simulink model "quad_equation_3d_porovnani_modelu_2024a"  (R2024a)
settings: Solver=FixedStepAuto  StartTime=0.0  StopTime=1  FixedStep=0.01  RelTol=1e-3
values from neighbouring files (symbols this model uses):
  b_moment = 0.01    [quad_param_3d.m]
  g = 9.81    [quad_param_3d.m]
  I = [Ixx, 0, 0 ... (first row only)    [quad_param_3d.m]
  Ixx = 1.1    [quad_param_3d.m]
  Iyy = 2.989    [quad_param_3d.m]
  Izz = 3.978    [quad_param_3d.m]
  k = 0.01    [quad_param_3d.m]
  k_thrust = 0.1    [quad_param_3d.m]
  L = 0.086    [quad_param_3d.m]
  M = 3.3    [quad_param_3d.m]
  Xinit = [0;0;0;0;0;0;0;0;0;0;0;0]    [quad_param_3d.m]
undefined symbols (not defined in the file or in its folder): Us, Xinit_matrix, Xinit_ss, Xs
libraries: simulink_extras x4
settings Model: Creator=Admin  LastModifiedBy=Admin

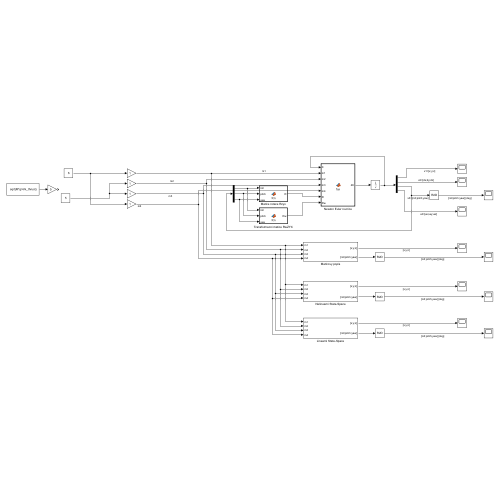
[thumbnail: Simulink's stored preview of the top-level diagram]
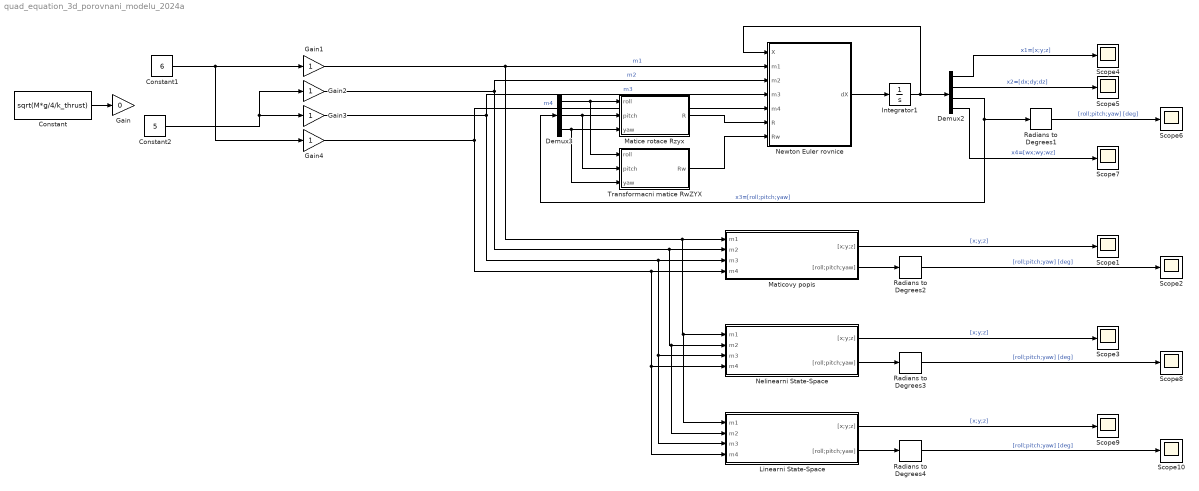
== system quad_equation_3d_porovnani_modelu_2024a ==
  Constant : Constant  Value=sqrt(M*g/4/k_thrust)
  Constant1 : Constant  Value=6
  Constant2 : Constant  Value=5
  Demux2 : Demux
  Demux3 : Demux  Outputs=3
  Gain : Gain  Gain=0
  Gain{1..4} (4 alike) : Gain
  Integrator1 : Integrator  InitialCondition=Xinit
  Linearni State-Space : Subsystem
  Matice rotace Rzyx : MATLAB Function  TreatAsAtomicUnit=on
  Maticovy popis : Subsystem
  Nelinearni State-Space : Subsystem
  Newton Euler rovnice : MATLAB Function  TreatAsAtomicUnit=on
  Radians to Degrees{1..4} (4 alike) : simulink_extras/Transformations/Radians to Degrees
  Scope{1..10} (10 alike) : Scope
  Transformacni matice RwZYX : MATLAB Function  TreatAsAtomicUnit=on
  wires:
  Demux2/1 -> Scope4/1  "x1=[x;y;z]"
  Demux3/2 -> Matice rotace Rzyx/2(pitch), Transformacni matice RwZYX/2(pitch)
  Demux3/3 -> Matice rotace Rzyx/3(yaw), Transformacni matice RwZYX/3(yaw)
  Gain4/1 -> Newton Euler rovnice/5(m4), Linearni State-Space/4(m4), Nelinearni State-Space/4(m4), Maticovy popis/4(m4)  "m4"
  Transformacni matice RwZYX/1(Rw) -> Newton Euler rovnice/7(Rw)
  Constant/1 -> Gain/1
  Gain1/1 -> Linearni State-Space/1(m1), Nelinearni State-Space/1(m1), Maticovy popis/1(m1), Newton Euler rovnice/2(m1)  "m1"
  Gain3/1 -> Newton Euler rovnice/4(m3), Linearni State-Space/3(m3), Nelinearni State-Space/3(m3), Maticovy popis/3(m3)  "m3"
  Demux2/4 -> Scope7/1  "x4=[wx;wy;wz]"
  Matice rotace Rzyx/1(R) -> Newton Euler rovnice/6(R)
  Demux2/3 -> Radians to Degrees1/1, Demux3/1  "x3=[roll;pitch;yaw]"
  Radians to Degrees1/1 -> Scope6/1  "[roll;pitch;yaw] [deg]"
  Demux3/1 -> Transformacni matice RwZYX/1(roll), Matice rotace Rzyx/1(roll)
  Newton Euler rovnice/1(dX) -> Integrator1/1
  Demux2/2 -> Scope5/1  "x2=[dx;dy;dz]"
  Gain2/1 -> Newton Euler rovnice/3(m2), Linearni State-Space/2(m2), Nelinearni State-Space/2(m2), Maticovy popis/2(m2)  "m2"
  Integrator1/1 -> Newton Euler rovnice/1(X), Demux2/1
  Maticovy popis/1("[x;y;z]") -> Scope1/1  "[x;y;z]"
  Radians to Degrees2/1 -> Scope2/1  "[roll;pitch;yaw] [deg]"
  Maticovy popis/2("[roll;pitch;yaw]") -> Radians to Degrees2/1
  Radians to Degrees3/1 -> Scope8/1  "[roll;pitch;yaw] [deg]"
  Nelinearni State-Space/1("[x;y;z]") -> Scope3/1  "[x;y;z]"
  Nelinearni State-Space/2("[roll;pitch;yaw]") -> Radians to Degrees3/1
  Radians to Degrees4/1 -> Scope10/1  "[roll;pitch;yaw] [deg]"
  Linearni State-Space/2("[roll;pitch;yaw]") -> Radians to Degrees4/1
  Linearni State-Space/1("[x;y;z]") -> Scope9/1  "[x;y;z]"
  Constant1/1 -> Gain4/1, Gain1/1
  Constant2/1 -> Gain3/1, Gain2/1

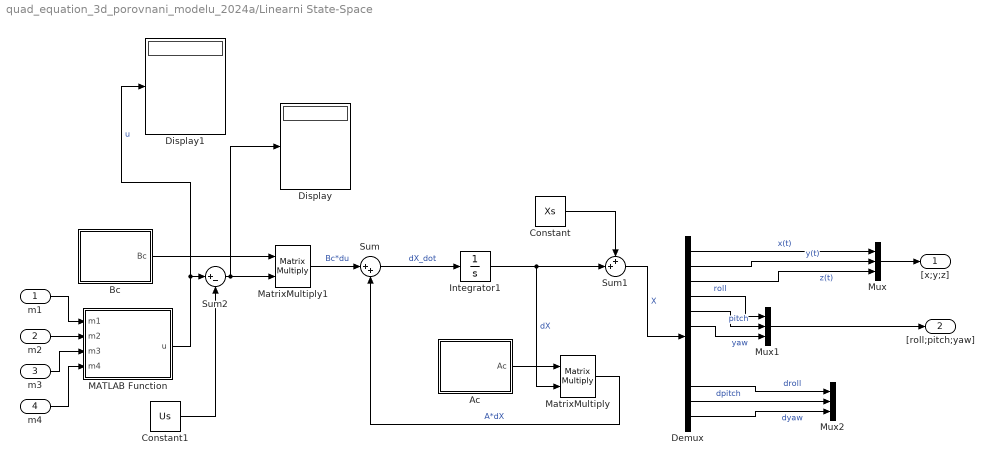
== system quad_equation_3d_porovnani_modelu_2024a/Linearni State-Space ==
  m1 : Inport
  m2 : Inport  Port=2
  m3 : Inport  Port=3
  m4 : Inport  Port=4
  Ac : MATLAB Function  TreatAsAtomicUnit=on
  Bc : MATLAB Function  TreatAsAtomicUnit=on
  Constant : Constant  Value=Xs
  Constant1 : Constant  Value=Us
  Demux : Demux  Outputs=12
  Display : Display
  Display1 : Display
  Integrator1 : Integrator  InitialCondition=Xinit_ss
  MATLAB Function : MATLAB Function  TreatAsAtomicUnit=on
  MatrixMultiply : Product  Multiplication=Matrix(*)
  MatrixMultiply1 : Product  Multiplication=Matrix(*)
  Mux : Mux  Inputs=3
  Mux1 : Mux  Inputs=3
  Mux2 : Mux  Inputs=3
  Sum : Sum  Inputs=|++
  Sum1 : Sum  Inputs=++|
  Sum2 : Sum  Inputs=|+-
  "[x;y;z]" : Outport
  "[roll;pitch;yaw]" : Outport  Port=2
  wires:
  MATLAB Function/1(u) -> Display1/1, Sum2/1  "u"
  m3/1 -> MATLAB Function/3(m3)
  m2/1 -> MATLAB Function/2(m2)
  m4/1 -> MATLAB Function/4(m4)
  m1/1 -> MATLAB Function/1(m1)
  Ac/1(Ac) -> MatrixMultiply/1
  Integrator1/1 -> Sum1/2, MatrixMultiply/2  "dX"
  Demux/1 -> Mux/1  "x(t)"
  Demux/2 -> Mux/2  "y(t)"
  Demux/3 -> Mux/3  "z(t)"
  Mux/1 -> "[x;y;z]"/1
  Demux/4 -> Mux1/1  "roll"
  Demux/5 -> Mux1/2  "pitch"
  Demux/6 -> Mux1/3  "yaw"
  Mux1/1 -> "[roll;pitch;yaw]"/1
  Demux/10 -> Mux2/1  "droll"
  Demux/11 -> Mux2/2  "dpitch"
  Demux/12 -> Mux2/3  "dyaw"
  Sum/1 -> Integrator1/1  "dX_dot"
  MatrixMultiply1/1 -> Sum/1  "Bc*du"
  MatrixMultiply/1 -> Sum/2  "A*dX"
  Bc/1(Bc) -> MatrixMultiply1/1
  Sum1/1 -> Demux/1  "X"
  Constant/1 -> Sum1/1
  Constant1/1 -> Sum2/2
  Sum2/1 -> Display/1, MatrixMultiply1/2

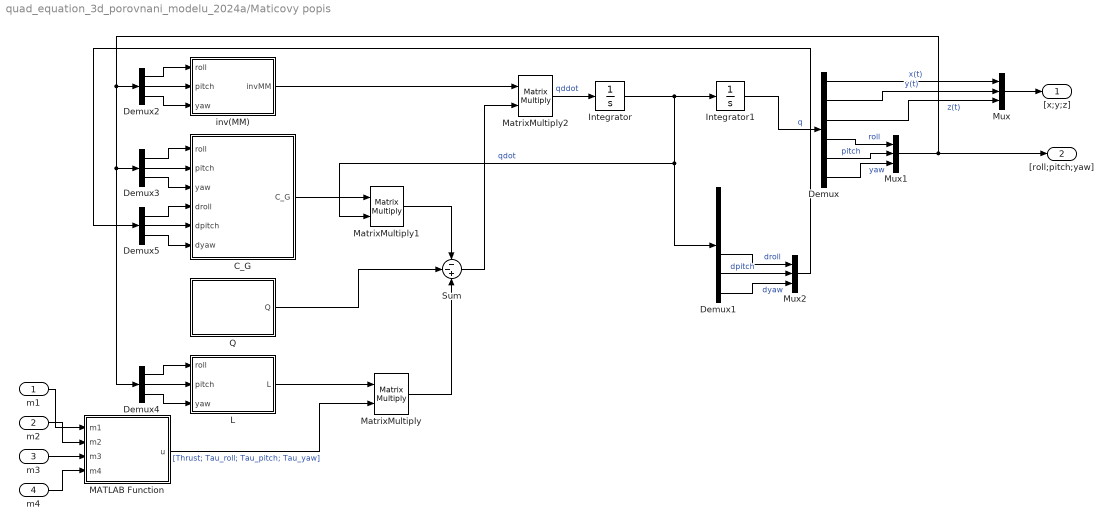
== system quad_equation_3d_porovnani_modelu_2024a/Maticovy popis ==
  m1 : Inport
  m2 : Inport  Port=2
  m3 : Inport  Port=3
  m4 : Inport  Port=4
  C_G : MATLAB Function  TreatAsAtomicUnit=on
  Demux : Demux  Outputs=6
  Demux1 : Demux  Outputs=6
  Demux{2..5} (4 alike) : Demux  Outputs=3
  Integrator : Integrator  InitialCondition=[0;0;0;0;0;0]
  Integrator1 : Integrator  InitialCondition=Xinit_matrix
  L : MATLAB Function  TreatAsAtomicUnit=on
  MATLAB Function : MATLAB Function  TreatAsAtomicUnit=on
  MatrixMultiply : Product  Multiplication=Matrix(*)
  MatrixMultiply1 : Product  Multiplication=Matrix(*)
  MatrixMultiply2 : Product  Multiplication=Matrix(*)
  Mux : Mux  Inputs=3
  Mux1 : Mux  Inputs=3
  Mux2 : Mux  Inputs=3
  Q : MATLAB Function  TreatAsAtomicUnit=on
  Sum : Sum  Inputs=--+
  inv(MM) : MATLAB Function  TreatAsAtomicUnit=on
  "[x;y;z]" : Outport
  "[roll;pitch;yaw]" : Outport  Port=2
  wires:
  inv(MM)/1(invMM) -> MatrixMultiply2/1
  L/1(L) -> MatrixMultiply/1
  MATLAB Function/1(u) -> MatrixMultiply/2  "[Thrust; Tau_roll; Tau_pitch; Tau_yaw]"
  m3/1 -> MATLAB Function/3(m3)
  m2/1 -> MATLAB Function/2(m2)
  m4/1 -> MATLAB Function/4(m4)
  MatrixMultiply/1 -> Sum/3
  m1/1 -> MATLAB Function/1(m1)
  Q/1(Q) -> Sum/2
  C_G/1(C_G) -> MatrixMultiply1/1
  MatrixMultiply1/1 -> Sum/1
  Sum/1 -> MatrixMultiply2/2
  MatrixMultiply2/1 -> Integrator/1  "qddot"
  Integrator/1 -> MatrixMultiply1/2, Demux1/1, Integrator1/1  "qdot"
  Integrator1/1 -> Demux/1  "q"
  Demux/1 -> Mux/1  "x(t)"
  Demux/2 -> Mux/2  "y(t)"
  Demux/3 -> Mux/3  "z(t)"
  Mux/1 -> "[x;y;z]"/1
  Demux/4 -> Mux1/1  "roll"
  Demux/5 -> Mux1/2  "pitch"
  Demux/6 -> Mux1/3  "yaw"
  Mux1/1 -> Demux4/1, Demux3/1, Demux2/1, "[roll;pitch;yaw]"/1
  Demux1/4 -> Mux2/1  "droll"
  Demux1/5 -> Mux2/2  "dpitch"
  Demux1/6 -> Mux2/3  "dyaw"
  Demux2/1 -> inv(MM)/1(roll)
  Demux2/2 -> inv(MM)/2(pitch)
  Demux2/3 -> inv(MM)/3(yaw)
  Demux3/2 -> C_G/2(pitch)
  Demux3/1 -> C_G/1(roll)
  Demux3/3 -> C_G/3(yaw)
  Demux4/2 -> L/2(pitch)
  Demux4/1 -> L/1(roll)
  Demux4/3 -> L/3(yaw)
  Demux5/2 -> C_G/5(dpitch)
  Demux5/1 -> C_G/4(droll)
  Demux5/3 -> C_G/6(dyaw)
  Mux2/1 -> Demux5/1

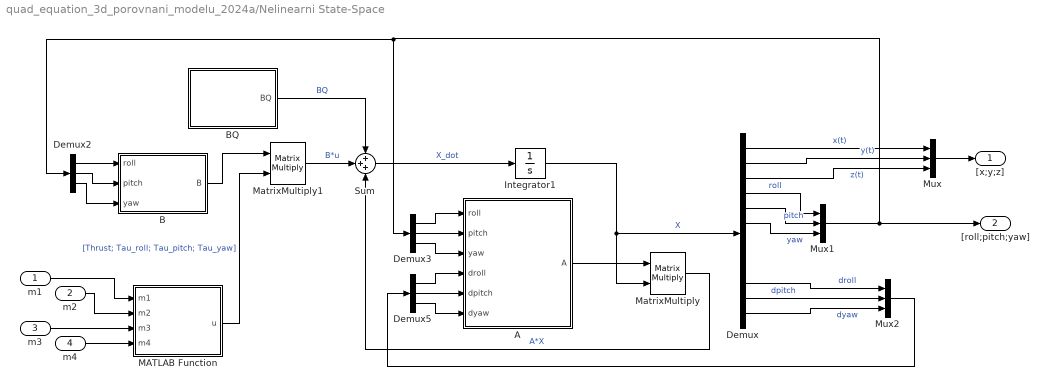
== system quad_equation_3d_porovnani_modelu_2024a/Nelinearni State-Space ==
  m1 : Inport
  m2 : Inport  Port=2
  m3 : Inport  Port=3
  m4 : Inport  Port=4
  A : MATLAB Function  TreatAsAtomicUnit=on
  B : MATLAB Function  TreatAsAtomicUnit=on
  BQ : MATLAB Function  TreatAsAtomicUnit=on
  Demux : Demux  Outputs=12
  Demux2 : Demux  Outputs=3
  Demux3 : Demux  Outputs=3
  Demux5 : Demux  Outputs=3
  Integrator1 : Integrator  InitialCondition=Xinit_ss
  MATLAB Function : MATLAB Function  TreatAsAtomicUnit=on
  MatrixMultiply : Product  Multiplication=Matrix(*)
  MatrixMultiply1 : Product  Multiplication=Matrix(*)
  Mux : Mux  Inputs=3
  Mux1 : Mux  Inputs=3
  Mux2 : Mux  Inputs=3
  Sum : Sum  Inputs=+++
  "[x;y;z]" : Outport
  "[roll;pitch;yaw]" : Outport  Port=2
  wires:
  MATLAB Function/1(u) -> MatrixMultiply1/2  "[Thrust; Tau_roll; Tau_pitch; Tau_yaw]"
  m3/1 -> MATLAB Function/3(m3)
  m2/1 -> MATLAB Function/2(m2)
  m4/1 -> MATLAB Function/4(m4)
  m1/1 -> MATLAB Function/1(m1)
  A/1(A) -> MatrixMultiply/1
  Integrator1/1 -> Demux/1, MatrixMultiply/2  "X"
  Demux/1 -> Mux/1  "x(t)"
  Demux/2 -> Mux/2  "y(t)"
  Demux/3 -> Mux/3  "z(t)"
  Mux/1 -> "[x;y;z]"/1
  Demux/4 -> Mux1/1  "roll"
  Demux/5 -> Mux1/2  "pitch"
  Demux/6 -> Mux1/3  "yaw"
  Mux1/1 -> Demux2/1, Demux3/1, "[roll;pitch;yaw]"/1
  Demux/10 -> Mux2/1  "droll"
  Demux/11 -> Mux2/2  "dpitch"
  Demux/12 -> Mux2/3  "dyaw"
  Demux2/1 -> B/1(roll)
  Demux2/2 -> B/2(pitch)
  Demux2/3 -> B/3(yaw)
  Demux3/2 -> A/2(pitch)
  Demux3/1 -> A/1(roll)
  Demux3/3 -> A/3(yaw)
  Demux5/2 -> A/5(dpitch)
  Demux5/1 -> A/4(droll)
  Demux5/3 -> A/6(dyaw)
  Sum/1 -> Integrator1/1  "X_dot"
  BQ/1(BQ) -> Sum/1  "BQ"
  MatrixMultiply1/1 -> Sum/2  "B*u"
  B/1(B) -> MatrixMultiply1/1
  MatrixMultiply/1 -> Sum/3  "A*X"
  Mux2/1 -> Demux5/1

== matlab function quad_equation_3d_porovnani_modelu_2024a/Maticovy popis/MATLAB Function ==
  data: u output; m1 input; m2 input; m3 input; m4 input; k_thrust parameter; b_moment parameter; L parameter
function u = fcn(m1, m2, m3, m4, k_thrust, b_moment, L)

Thrust = k_thrust*(m1^2 + m2^2 + m3^2 + m4^2);
Tau_roll = L*k_thrust*(m1^2 + m4^2 - m2^2 - m3^2);
Tau_pitch = L*k_thrust*(m4^2 + m3^2 - m1^2 - m2^2);
Tau_yaw = b_moment*(m1^2 + m3^2 - m2^2 - m4^2);

u = [Thrust; Tau_roll; Tau_pitch; Tau_yaw];

== matlab function quad_equation_3d_porovnani_modelu_2024a/Nelinearni State-Space/A ==
  data: roll input; A output; pitch input; yaw input; droll input; dpitch input; dyaw input; k parameter; Ixx parameter; Iyy parameter; Izz parameter; M parameter
function A = fcn(roll, pitch, yaw, droll, dpitch, dyaw, k, Ixx, Iyy, Izz, M)
% Matice dynamiky A

phi_t = roll;
theta_t = pitch;
psi_t = yaw;

phi_dot_t = droll;
theta_dot_t = dpitch;
psi_dot_t = dyaw;

A = [
0, 0, 0, 0, 0, 0,    1,    0,    0,                                                                                                                                                                                                                                                                                                                                                                                                                                                                                                                               0,                                                                                                                                                                                                                                                                                                                                                                                                                                                                                                                                                                                                                                    0,                                                                                                                                                                                                                                                                                                                                                                                                                                                                                         0;
0, 0, 0, 0, 0, 0,    0,    1,    0,                                                                                                                                                                                                                                                                                                                                                                                                                                                                                                                               0,                                                                                                                                                                                                                                                                                                                                                                                                                                                                                                                                                                                                                                    0,                                                                                                                                                                                                                                                                                                                                                                                                                                                                                         0;
0, 0, 0, 0, 0, 0,    0,    0,    1,                                                                                                                                                                                                                                                                                                                                                                                                                                                                                                                               0,                                                                                                                                                                                                                                                                                                                                                                                                                                                                                                                                                                                                                                    0,                                                                                                                                                                                                                                                                                                                                                                                                                                                                                         0;
0, 0, 0, 0, 0, 0,    0,    0,    0,                                                                                                                                                                                                                                                                                                                                                                                                                                                                                                                               1,                                                                                                                                                                                                                                                                                                                                                                                                                                                                                                                                                                                                                                    0,                                                                                                                                                                                                                                                                                                                                                                                                                                                                                         0;
0, 0, 0, 0, 0, 0,    0,    0,    0,                                                                                                                                                                                                                                                                                                                                                                                                                                                                                                                               0,                                                                                                                                                                                                                                                                                                                                                                                                                                                                                                                                                                                                                                    1,                                                                                                                                                                                                                                                                                                                                                                                                                                                                                         0;
0, 0, 0, 0, 0, 0,    0,    0,    0,                                                                                                                                                                                                                                                                                                                                                                                                                                                                                                                               0,                                                                                                                                                                                                                                                                                                                                                                                                                                                                                                                                                                                                                                    0,                                                                                                                                                                                                                                                                                                                                                                                                                                                                                         1;
0, 0, 0, 0, 0, 0, -k/M,    0,    0,                                                                                                                                                                                                                                                                                                                                                                                                                                                                                                                               0,                                                                                                                                                                                                                                                                                                                                                                                                                                                                                                                                                                                                                                    0,                                                                                                                                                                                                                                                                                                                                                                                                                                                                                         0;
0, 0, 0, 0, 0, 0,    0, -k/M,    0,                                                                                                                                                                                                                                                                                                                                                                                                                                                                                                                               0,                                                                                                                                                                                                                                                                                                                                                                                                                                                                                                                                                                                                                                    0,                                                                                                                                                                                                                                                                                                                                                                                                                                                                                         0;
0, 0, 0, 0, 0, 0,    0,    0, -k/M,                                                                                                                                                                                                                                                                                                                                                                                                                                                                                                                               0,                                                                                                                                                                                                                                                                                                                                                                                                                                                                                                                                                                                                                                    0,                                                                                                                                                                                                                                                                                                                                                                                                                                                                                         0;
0, 0, 0, 0, 0, 0,    0,    0,    0, (cos(phi_t)*sin(theta_t)*(psi_dot_t*(Ixx*cos(theta_t)*sin(phi_t) - Iyy*cos(theta_t)*sin(phi_t) + Izz*cos(theta_t)*sin(phi_t)) + theta_dot_t*(Ixx*cos(phi_t) - Iyy*cos(phi_t) + Izz*cos(phi_t))))/(Izz*(cos(theta_t)*cos(phi_t)^2 + cos(theta_t)*sin(phi_t)^2)) - (sin(phi_t)*sin(theta_t)*(psi_dot_t*(Ixx*cos(phi_t)*cos(theta_t) + Iyy*cos(phi_t)*cos(theta_t) - Izz*cos(phi_t)*cos(theta_t)) - theta_dot_t*(Ixx*sin(phi_t) + Iyy*sin(phi_t) - Izz*sin(phi_t))))/(Iyy*(cos(theta_t)*cos(phi_t)^2 + cos(theta_t)*sin(phi_t)^2)), (psi_dot_t*(Ixx*cos(theta_t) + Iyy*cos(phi_t)^2*cos(theta_t) - Izz*cos(phi_t)^2*cos(theta_t) - Iyy*cos(theta_t)*sin(phi_t)^2 + Izz*cos(theta_t)*sin(phi_t)^2) - theta_dot_t*(Iyy*cos(phi_t)*sin(phi_t) - Izz*cos(phi_t)*sin(phi_t)))/Ixx + (psi_dot_t*cos(phi_t)*sin(theta_t)*(Iyy*cos(phi_t)*sin(theta_t) - Ixx*cos(phi_t)*sin(theta_t) + Izz*cos(phi_t)*sin(theta_t)))/(Izz*(cos(theta_t)*cos(phi_t)^2 + cos(theta_t)*sin(phi_t)^2)) + (psi_dot_t*sin(phi_t)*sin(theta_t)*(Iyy*sin(phi_t)*sin(theta_t) - Ixx*sin(phi_t)*sin(theta_t) + Izz*sin(phi_t)*sin(theta_t)))/(Iyy*(cos(theta_t)*cos(phi_t)^2 + cos(theta_t)*sin(phi_t)^2)), (psi_dot_t*(Iyy*cos(phi_t)*cos(theta_t)^2*sin(phi_t) - Izz*cos(phi_t)*cos(theta_t)^2*sin(phi_t)))/Ixx + (psi_dot_t*sin(phi_t)*sin(theta_t)*(Ixx*cos(phi_t)*cos(theta_t)*sin(theta_t) - Izz*cos(phi_t)*cos(theta_t)*sin(theta_t)))/(Iyy*(cos(theta_t)*cos(phi_t)^2 + cos(theta_t)*sin(phi_t)^2)) - (psi_dot_t*cos(phi_t)*sin(theta_t)*(Ixx*cos(theta_t)*sin(phi_t)*sin(theta_t) - Iyy*cos(theta_t)*sin(phi_t)*sin(theta_t)))/(Izz*(cos(theta_t)*cos(phi_t)^2 + cos(theta_t)*sin(phi_t)^2));
0, 0, 0, 0, 0, 0,    0,    0,    0,                                                                             - (cos(phi_t)*(psi_dot_t*(Ixx*cos(phi_t)*cos(theta_t) + Iyy*cos(phi_t)*cos(theta_t) - Izz*cos(phi_t)*cos(theta_t)) - theta_dot_t*(Ixx*sin(phi_t) + Iyy*sin(phi_t) - Izz*sin(phi_t))))/(Iyy*(cos(phi_t)^2 + sin(phi_t)^2)) - (sin(phi_t)*(psi_dot_t*(Ixx*cos(theta_t)*sin(phi_t) - Iyy*cos(theta_t)*sin(phi_t) + Izz*cos(theta_t)*sin(phi_t)) + theta_dot_t*(Ixx*cos(phi_t) - Iyy*cos(phi_t) + Izz*cos(phi_t))))/(Izz*(cos(phi_t)^2 + sin(phi_t)^2)),                                                                                                                                                                                                                                                                                                                          (psi_dot_t*cos(phi_t)*(Iyy*sin(phi_t)*sin(theta_t) - Ixx*sin(phi_t)*sin(theta_t) + Izz*sin(phi_t)*sin(theta_t)))/(Iyy*(cos(phi_t)^2 + sin(phi_t)^2)) - (psi_dot_t*sin(phi_t)*(Iyy*cos(phi_t)*sin(theta_t) - Ixx*cos(phi_t)*sin(theta_t) + Izz*cos(phi_t)*sin(theta_t)))/(Izz*(cos(phi_t)^2 + sin(phi_t)^2)),                                                                                                                                                                                       (psi_dot_t*cos(phi_t)*(Ixx*cos(phi_t)*cos(theta_t)*sin(theta_t) - Izz*cos(phi_t)*cos(theta_t)*sin(theta_t)))/(Iyy*(cos(phi_t)^2 + sin(phi_t)^2)) + (psi_dot_t*sin(phi_t)*(Ixx*cos(theta_t)*sin(phi_t)*sin(theta_t) - Iyy*cos(theta_t)*sin(phi_t)*sin(theta_t)))/(Izz*(cos(phi_t)^2 + sin(phi_t)^2));
0, 0, 0, 0, 0, 0,    0,    0,    0,                           (cos(phi_t)*(psi_dot_t*(Ixx*cos(theta_t)*sin(phi_t) - Iyy*cos(theta_t)*sin(phi_t) + Izz*cos(theta_t)*sin(phi_t)) + theta_dot_t*(Ixx*cos(phi_t) - Iyy*cos(phi_t) + Izz*cos(phi_t))))/(Izz*(cos(theta_t)*cos(phi_t)^2 + cos(theta_t)*sin(phi_t)^2)) - (sin(phi_t)*(psi_dot_t*(Ixx*cos(phi_t)*cos(theta_t) + Iyy*cos(phi_t)*cos(theta_t) - Izz*cos(phi_t)*cos(theta_t)) - theta_dot_t*(Ixx*sin(phi_t) + Iyy*sin(phi_t) - Izz*sin(phi_t))))/(Iyy*(cos(theta_t)*cos(phi_t)^2 + cos(theta_t)*sin(phi_t)^2)),                                                                                                                                                                                                                                                                      (psi_dot_t*cos(phi_t)*(Iyy*cos(phi_t)*sin(theta_t) - Ixx*cos(phi_t)*sin(theta_t) + Izz*cos(phi_t)*sin(theta_t)))/(Izz*(cos(theta_t)*cos(phi_t)^2 + cos(theta_t)*sin(phi_t)^2)) + (psi_dot_t*sin(phi_t)*(Iyy*sin(phi_t)*sin(theta_t) - Ixx*sin(phi_t)*sin(theta_t) + Izz*sin(phi_t)*sin(theta_t)))/(Iyy*(cos(theta_t)*cos(phi_t)^2 + cos(theta_t)*sin(phi_t)^2)),                                                                                                                                   (psi_dot_t*sin(phi_t)*(Ixx*cos(phi_t)*cos(theta_t)*sin(theta_t) - Izz*cos(phi_t)*cos(theta_t)*sin(theta_t)))/(Iyy*(cos(theta_t)*cos(phi_t)^2 + cos(theta_t)*sin(phi_t)^2)) - (psi_dot_t*cos(phi_t)*(Ixx*cos(theta_t)*sin(phi_t)*sin(theta_t) - Iyy*cos(theta_t)*sin(phi_t)*sin(theta_t)))/(Izz*(cos(theta_t)*cos(phi_t)^2 + cos(theta_t)*sin(phi_t)^2))];

== matlab function quad_equation_3d_porovnani_modelu_2024a/Nelinearni State-Space/BQ ==
  data: BQ output; g parameter
function BQ = fcn(g)
% Matice vstupu tihy
BQ = [0 0 0 0 0 0 0 0 -g 0 0 0]';

== matlab function quad_equation_3d_porovnani_modelu_2024a/Nelinearni State-Space/MATLAB Function ==
  data: u output; m1 input; m2 input; m3 input; m4 input; k_thrust parameter; b_moment parameter; L parameter
function u = fcn(m1, m2, m3, m4, k_thrust, b_moment, L)

Thrust = k_thrust*(m1^2 + m2^2 + m3^2 + m4^2);
Tau_roll = L*k_thrust*(m1^2 + m4^2 - m2^2 - m3^2);
Tau_pitch = L*k_thrust*(m4^2 + m3^2 - m1^2 - m2^2);
Tau_yaw = b_moment*(m1^2 + m3^2 - m2^2 - m4^2);

u = [Thrust; Tau_roll; Tau_pitch; Tau_yaw];

== matlab function quad_equation_3d_porovnani_modelu_2024a/Linearni State-Space/Bc ==
  data: M parameter; Bc output; Ixx parameter; Iyy parameter; Izz parameter
function Bc = fcn(M, Ixx, Iyy, Izz)
% Matice Ac linearizovana

Bc = [
  0,     0,     0,     0;
  0,     0,     0,     0;
  0,     0,     0,     0;
  0,     0,     0,     0;
  0,     0,     0,     0;
  0,     0,     0,     0;
  0,     0,     0,     0;
  0,     0,     0,     0;
1/M,     0,     0,     0;
  0, 1/Ixx,     0,     0;
  0,     0, 1/Iyy,     0;
  0,     0,     0, 1/Izz];

== matlab function quad_equation_3d_porovnani_modelu_2024a/Nelinearni State-Space/B ==
  data: roll input; B output; pitch input; yaw input; M parameter; Ixx parameter; Iyy parameter; Izz parameter
function B = fcn(roll, pitch, yaw, M, Ixx, Iyy, Izz)
% Matice vstupu do soustavy kvadrokoptery

phi_t = roll;
theta_t = pitch;
psi_t = yaw;

B = [
                                                              0,     0,                                                                          0,                                                                          0;
                                                              0,     0,                                                                          0,                                                                          0;
                                                              0,     0,                                                                          0,                                                                          0;
                                                              0,     0,                                                                          0,                                                                          0;
                                                              0,     0,                                                                          0,                                                                          0;
                                                              0,     0,                                                                          0,                                                                          0;
 (sin(phi_t)*sin(psi_t) + cos(phi_t)*cos(psi_t)*sin(theta_t))/M,     0,                                                                          0,                                                                          0;
-(cos(psi_t)*sin(phi_t) - cos(phi_t)*sin(psi_t)*sin(theta_t))/M,     0,                                                                          0,                                                                          0;
                                    (cos(phi_t)*cos(theta_t))/M,     0,                                                                          0,                                                                          0;
                                                              0, 1/Ixx, (sin(phi_t)*sin(theta_t))/(Iyy*cos(theta_t)*(cos(phi_t)^2 + sin(phi_t)^2)), (cos(phi_t)*sin(theta_t))/(Izz*cos(theta_t)*(cos(phi_t)^2 + sin(phi_t)^2));
                                                              0,     0,                             cos(phi_t)/(Iyy*(cos(phi_t)^2 + sin(phi_t)^2)),                            -sin(phi_t)/(Izz*(cos(phi_t)^2 + sin(phi_t)^2));
                                                              0,     0,                sin(phi_t)/(Iyy*cos(theta_t)*(cos(phi_t)^2 + sin(phi_t)^2)),                cos(phi_t)/(Izz*cos(theta_t)*(cos(phi_t)^2 + sin(phi_t)^2))];

== matlab function quad_equation_3d_porovnani_modelu_2024a/Linearni State-Space/MATLAB Function ==
  data: u output; m1 input; m2 input; m3 input; m4 input; k_thrust parameter; b_moment parameter; L parameter
function u = fcn(m1, m2, m3, m4, k_thrust, b_moment, L)

Thrust = k_thrust*(m1^2 + m2^2 + m3^2 + m4^2);
Tau_roll = L*k_thrust*(m1^2 + m4^2 - m2^2 - m3^2);
Tau_pitch = L*k_thrust*(m4^2 + m3^2 - m1^2 - m2^2);
Tau_yaw = b_moment*(m1^2 + m3^2 - m2^2 - m4^2);

u = [Thrust; Tau_roll; Tau_pitch; Tau_yaw];

== matlab function quad_equation_3d_porovnani_modelu_2024a/Linearni State-Space/Ac ==
  data: Ac output; k parameter; g parameter; M parameter
function Ac = fcn(k, g, M)
% Matice Ac linearizovana

Ac = [ 
0, 0, 0,  0, 0, 0,    1,    0,    0, 0, 0, 0;
0, 0, 0,  0, 0, 0,    0,    1,    0, 0, 0, 0;
0, 0, 0,  0, 0, 0,    0,    0,    1, 0, 0, 0;
0, 0, 0,  0, 0, 0,    0,    0,    0, 1, 0, 0;
0, 0, 0,  0, 0, 0,    0,    0,    0, 0, 1, 0;
0, 0, 0,  0, 0, 0,    0,    0,    0, 0, 0, 1;
0, 0, 0,  0, g, 0, -k/M,    0,    0, 0, 0, 0;
0, 0, 0, -g, 0, 0,    0, -k/M,    0, 0, 0, 0;
0, 0, 0,  0, 0, 0,    0,    0, -k/M, 0, 0, 0;
0, 0, 0,  0, 0, 0,    0,    0,    0, 0, 0, 0;
0, 0, 0,  0, 0, 0,    0,    0,    0, 0, 0, 0;
0, 0, 0,  0, 0, 0,    0,    0,    0, 0, 0, 0];

== matlab function quad_equation_3d_porovnani_modelu_2024a/Maticovy popis/C_G ==
  data: roll input; C_G output; pitch input; yaw input; droll input; dpitch input; dyaw input; k parameter; Ixx parameter; Iyy parameter; Izz parameter
function C_G = fcn(roll, pitch, yaw, droll, dpitch, dyaw, k, Ixx, Iyy, Izz)
% Matice Coriolisovych sil a odporu vzduchu

phi_t = roll;
theta_t = pitch;
psi_t = yaw;

phi_dot_t = droll;
theta_dot_t = dpitch;
psi_dot_t = dyaw;


C_G = [
k, 0, 0,                                                                                                                                                                      0,                                                                                                                                                                                                                                  0,                                                                                                0;
0, k, 0,                                                                                                                                                                      0,                                                                                                                                                                                                                                  0,                                                                                                0;
0, 0, k,                                                                                                                                                                      0,                                                                                                                                                                                                                                  0,                                                                                                0;
0, 0, 0,                                                                                                                                                                      0, theta_dot_t*(Iyy*cos(phi_t)*sin(phi_t) - Izz*cos(phi_t)*sin(phi_t)) - psi_dot_t*(Ixx*cos(theta_t) + Iyy*cos(phi_t)^2*cos(theta_t) - Izz*cos(phi_t)^2*cos(theta_t) - Iyy*cos(theta_t)*sin(phi_t)^2 + Izz*cos(theta_t)*sin(phi_t)^2), -psi_dot_t*(Iyy*cos(phi_t)*cos(theta_t)^2*sin(phi_t) - Izz*cos(phi_t)*cos(theta_t)^2*sin(phi_t));
0, 0, 0,   psi_dot_t*(Ixx*cos(phi_t)*cos(theta_t) + Iyy*cos(phi_t)*cos(theta_t) - Izz*cos(phi_t)*cos(theta_t)) - theta_dot_t*(Ixx*sin(phi_t) + Iyy*sin(phi_t) - Izz*sin(phi_t)),                                                                                                                               -psi_dot_t*(Iyy*sin(phi_t)*sin(theta_t) - Ixx*sin(phi_t)*sin(theta_t) + Izz*sin(phi_t)*sin(theta_t)), -psi_dot_t*(Ixx*cos(phi_t)*cos(theta_t)*sin(theta_t) - Izz*cos(phi_t)*cos(theta_t)*sin(theta_t));
0, 0, 0, - psi_dot_t*(Ixx*cos(theta_t)*sin(phi_t) - Iyy*cos(theta_t)*sin(phi_t) + Izz*cos(theta_t)*sin(phi_t)) - theta_dot_t*(Ixx*cos(phi_t) - Iyy*cos(phi_t) + Izz*cos(phi_t)),                                                                                                                               -psi_dot_t*(Iyy*cos(phi_t)*sin(theta_t) - Ixx*cos(phi_t)*sin(theta_t) + Izz*cos(phi_t)*sin(theta_t)),  psi_dot_t*(Ixx*cos(theta_t)*sin(phi_t)*sin(theta_t) - Iyy*cos(theta_t)*sin(phi_t)*sin(theta_t))];

== matlab function quad_equation_3d_porovnani_modelu_2024a/Maticovy popis/inv(MM) ==
  data: roll input; invMM output; pitch input; yaw input; M parameter; Ixx parameter; Iyy parameter; Izz parameter
function invMM = fcn(roll, pitch, yaw, M, Ixx, Iyy, Izz)
% Matice hmotnosti a setrvacnosti

phi_t = roll;
theta_t = pitch;
psi_t = yaw;

MM = [
M, 0, 0,   0,               0,                           0;
0, M, 0,   0,               0,                           0;
0, 0, M,   0,               0,                           0;
0, 0, 0, Ixx,               0,           -Ixx*sin(theta_t);
0, 0, 0,   0,  Iyy*cos(phi_t), Iyy*cos(theta_t)*sin(phi_t);
0, 0, 0,   0, -Izz*sin(phi_t), Izz*cos(phi_t)*cos(theta_t)];

invMM = inv(MM);

== matlab function quad_equation_3d_porovnani_modelu_2024a/Maticovy popis/Q ==
  data: M parameter; Q output; g parameter
function Q = fcn(M, g)
% Matice tihovych sil
Q = [0 0 M*g 0 0 0]';

== matlab function quad_equation_3d_porovnani_modelu_2024a/Matice rotace Rzyx ==
  data: roll input; R output; pitch input; yaw input
function R = fcn(roll, pitch, yaw)
% Prepocet matice rotace R=Rx*Ry*Rz

R_x = [1, 0, 0; 
       0, cos(roll), -sin(roll);
       0, sin(roll), cos(roll)];

R_y = [cos(pitch), 0, sin(pitch); 
       0, 1, 0; 
      -sin(pitch), 0, cos(pitch)];

R_z = [cos(yaw), -sin(yaw), 0; 
       sin(yaw), cos(yaw), 0; 
       0, 0, 1];

R = R_z * R_y * R_x;

== matlab function quad_equation_3d_porovnani_modelu_2024a/Newton Euler rovnice ==
  data: X input; m1 input; dX output; m2 input; m3 input; m4 input; R input; Rw input; k_thrust parameter; k parameter; I parameter; g parameter; M parameter; L parameter; b_moment parameter
function dX  = fcn(X, m1, m2, m3, m4, R, Rw, k_thrust, k, I, g, M, L, b_moment)
% m1, m2, m3, m4 jsou odpovidajici uhlove rychlosti rotoru
% Stavovy popis
% x1 - pozice dronu v prostoru, [x;y;z]
% x2 - linearni rychlost, [dx;dy;dz]
% x3 - Eulerove uhly, [roll;pitch;yaw]
% x4 - vektor uhlovych rychlosti, [wx;wy;wz]
x1 = X(1:3);
x2 = X(4:6);
x3 = X(7:9);
x4 = X(10:12);

Thrust = k_thrust*(m1^2 + m2^2 + m3^2 + m4^2); % tahova sila v soustave tela
Friction = -k * x2; % odporova sila v soustave sveta
Tau_roll = L*k_thrust*(m1^2 + m4^2 - m2^2 - m3^2);
Tau_pitch = L*k_thrust*(m4^2 + m3^2 - m1^2 - m2^2);
Tau_yaw = b_moment*(m1^2 + m3^2 - m2^2 - m4^2);

dx1 = x2;
dx2 = [0; 0; -g] + 1/M*R*[0; 0; Thrust] + 1/M*Friction;
dx3 = Rw \ x4;
dx4 = I\( [Tau_roll; Tau_pitch; Tau_yaw] -  cross( x4, (I*x4) ) );

dX = [dx1; dx2; dx3; dx4];

== matlab function quad_equation_3d_porovnani_modelu_2024a/Transformacni matice RwZYX ==
  data: roll input; Rw output; pitch input; yaw input
function Rw = fcn(roll, pitch, yaw)
% Prepocet matice pro transformace derivaci Eulerovych uhlu 
% do uhlove rychlosti v soustave tela ?
Rw = [1, 0, -sin(pitch);
      0, cos(roll), cos(pitch)*sin(roll);
      0 -sin(roll), cos(pitch)*cos(roll)];

== matlab function quad_equation_3d_porovnani_modelu_2024a/Maticovy popis/L ==
  data: roll input; L output; pitch input; yaw input
function L = fcn(roll, pitch, yaw)
% Matice vah vstupu

phi_t = roll;
theta_t = pitch;
psi_t = yaw;

L = [
sin(phi_t)*sin(psi_t) + cos(phi_t)*cos(psi_t)*sin(theta_t), 0, 0, 0;
cos(phi_t)*sin(psi_t)*sin(theta_t) - cos(psi_t)*sin(phi_t), 0, 0, 0;
                                   cos(phi_t)*cos(theta_t), 0, 0, 0;
                                                         0, 1, 0, 0;
                                                         0, 0, 1, 0;
                                                         0, 0, 0, 1];
